simulink model "proxy"  (R2017b)
settings: Solver=ode3  StartTime=0.0  StopTime=inf  FixedStep=0.01  RelTol=1e-3  EnableMultiTasking=on
model workspace (MAT data in the model file):
  SL_ROS_VariableLengthArrays_MaxSizes.CommonInfo.ArrayTruncateAction = 'EmitWarning'
  SL_ROS_VariableLengthArrays_MaxSizes.MsgTypeMap = containers.Map
  SL_ROS_VariableLengthArrays_MaxSizes.MsgTypeMap.serialization.keys = {'std_msgs/Float32MultiArray'}
  SL_ROS_VariableLengthArrays_MaxSizes.MsgTypeMap.serialization.values{1}.PropertyName = 'Data'
  SL_ROS_VariableLengthArrays_MaxSizes.MsgTypeMap.serialization.values{1}.DataType = 'single'
  SL_ROS_VariableLengthArrays_MaxSizes.MsgTypeMap.serialization.values{1}.MaxLength = 2
  SL_ROS_VariableLengthArrays_MaxSizes.MsgTypeMap.serialization.uniformity = 0
  SL_ROS_VariableLengthArrays_MaxSizes.MsgTypeMap.serialization.keyType = 'char'
  SL_ROS_VariableLengthArrays_MaxSizes.MsgTypeMap.serialization.valueType = 'any'
values from neighbouring files (symbols this model uses):
  filt = c2d(filt,sampleTime)    [Connect.m]
libraries: robotlib x8, simulink x6, simulink_extras x3, dspnetwork x3, etargetslib x2, xpcutilitieslib x1
(part 1 of 4)
settings Model: Creator=Centauro  LastModifiedBy=BCI-USER
settings DataIOCC: LimitDataPoints=on  SaveFormat=Array
settings OptimizationCC: PassReuseOutputArgsThreshold=0  MaxStackSize=64
settings DebuggingCC: ParameterTunabilityLossMsg=error  SFUnexpectedBacktrackingDiag=warning  SFNoUnconditionalDefaultTransitionDiag=warning  SFExecutionAtInitializationDiag=none
settings HardwareCC: ProdBitPerPointer=32  ProdBitPerSizeT=32  ProdBitPerPtrDiffT=32  ProdLargestAtomicFloat=None  ProdIntDivRoundTo=Undefined  ProdEndianess=Unspecified  ProdWordSize=32  ProdHWDeviceType=Generic->Unspecified (assume 32-bit Generic)  UseEmbeddedCoderFeatures=off
settings ModelReferenceCC: PropagateSignalLabelsOutOfModel=off
settings SFSimCC: MATLABDynamicMemAlloc=off
settings RTWCC: SystemTargetFile=ert.tlc  HardwareBoard=Robot Operating System (ROS)  TemplateMakefile=ert_default_tmf  GenerateReport=on  Toolchain=Catkin  LaunchReport=on  TargetLang=C++
settings CodeAppCC: ForceParamTrailComments=on  OperatorAnnotations=on
settings ERTTargetCC: ERTCustomFileBanners=off  SupportContinuousTime=on  SupportNonInlinedSFcns=on  RemoveResetFunc=off  ModelStepFunctionPrototypeControlCompliant=off
settings ConfigComp: CovMetricSettings=dw  CovHtmlReporting=on  CovSaveCumulativeToWorkspaceVar=on  CovSaveSingleToWorkspaceVar=on  CovExternalEMLEnable=off

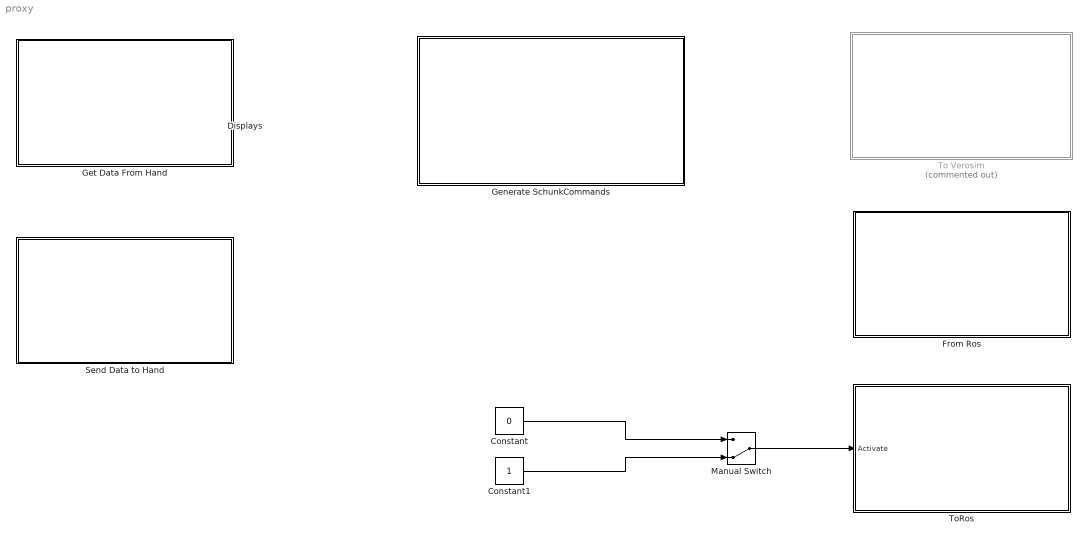
== system proxy ==
  Constant : Constant  Value=0  OutDataTypeStr=boolean
  Constant1 : Constant  OutDataTypeStr=boolean
  "Displays " : Subsystem
  From Ros : Subsystem
  "Generate SchunkCommands " : Subsystem
  Get Data From Hand : Subsystem
  Manual Switch : ManualSwitch  CurrentSetting=0
  Send Data to Hand : Subsystem
  To Verosim : Subsystem  Commented=on
  ToRos : Subsystem
  wires:
  Manual Switch/1 -> ToRos/1(Activate)
  Constant/1 -> Manual Switch/1
  Constant1/1 -> Manual Switch/2

== system proxy/Displays  ==
  Display{,1..3} (4 alike) : Display
  wires:
  [Forces] -> Display1/1
  [RotativePot] -> Display3/1
  [Header] -> Display/1
  [MotorsPot] -> Display2/1

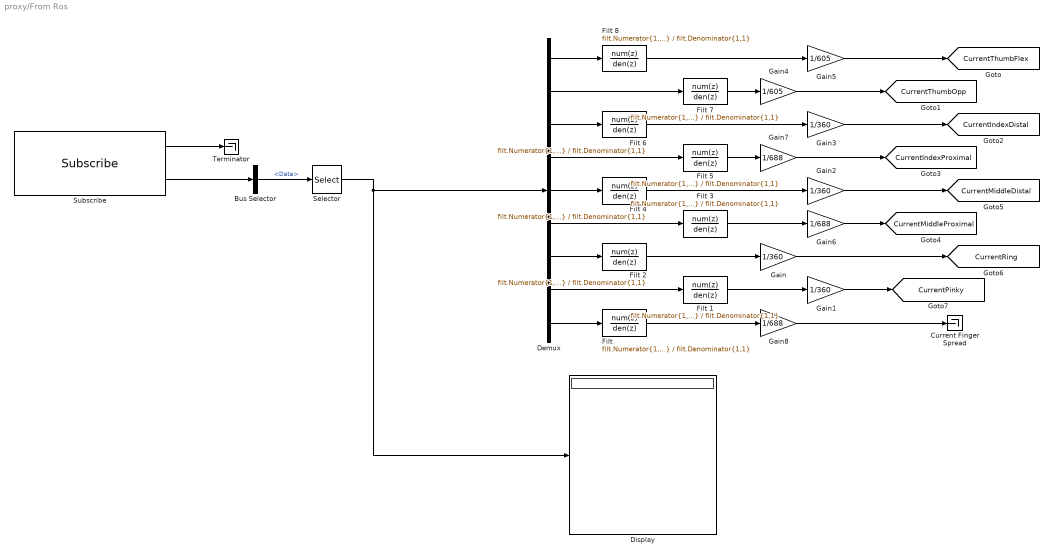
== system proxy/From Ros ==
  Bus Selector : BusSelector  OutputSignals=Data
  Current Finger Spread : Terminator
  Demux : Demux  Outputs=9
  Display : Display
  Filt {,1..8} (9 alike) : DiscreteTransferFcn  Numerator=filt.Numerator{1,1}  Denominator=filt.Denominator{1,1}  SampleTime=0.01
  Gain{,1..3} (4 alike) : Gain  Gain=1/360
  Gain4 : Gain  Gain=1/605
  Gain5 : Gain  Gain=1/605
  Gain6 : Gain  Gain=1/688
  Gain7 : Gain  Gain=1/688
  Gain8 : Gain  Gain=1/688
  Selector : Selector  IndexOptions=Index vector (dialog)  Indices=[1 2 3 4 5 6 7 8 9]  OutputSizes=1
  Subscribe : robotlib/Subscribe  SourceLibraryInfo=This block requires Robotics System Toolbox  topicSource=Select from ROS network  topic=/svh_controller/channel_currents  messageType=std_msgs/Float64MultiArray  sampleTime=0.01  messageQueueLength=1
      settings: SourceProductBaseCode=RO
  Terminator : Terminator
  tag scope: CurrentIndexDistal=global, CurrentIndexProximal=global, CurrentMiddleDistal=global, CurrentMiddleProximal=global, CurrentPinky=global, CurrentRing=global, CurrentThumbFlex=global, CurrentThumbOpp=global
  wires:
  Subscribe/1 -> Terminator/1
  Subscribe/2 -> Bus Selector/1
  Bus Selector/1 -> Selector/1  "<Data>"
  Selector/1 -> Demux/1, Display/1
  Demux/1 -> Filt 8/1
  Demux/2 -> Filt 7/1
  Demux/3 -> Filt 6/1
  Demux/4 -> Filt 5/1
  Demux/6 -> Filt 3/1
  Demux/5 -> Filt 4/1
  Demux/7 -> Filt 2/1
  Demux/8 -> Filt 1/1
  Demux/9 -> "Filt "/1
  "Filt "/1 -> Gain8/1
  Filt 1/1 -> Gain1/1
  Filt 2/1 -> Gain/1
  Filt 4/1 -> Gain2/1
  Filt 5/1 -> Gain7/1
  Filt 6/1 -> Gain3/1
  Filt 7/1 -> Gain4/1
  Filt 8/1 -> Gain5/1
  Gain1/1 -> [CurrentPinky]
  Gain/1 -> [CurrentRing]
  Filt 3/1 -> Gain6/1
  Gain2/1 -> [CurrentMiddleDistal]
  Gain3/1 -> [CurrentIndexDistal]
  Gain5/1 -> [CurrentThumbFlex]
  Gain4/1 -> [CurrentThumbOpp]
  Gain7/1 -> [CurrentIndexProximal]
  Gain6/1 -> [CurrentMiddleProximal]
  Gain8/1 -> Current Finger Spread/1

== system proxy/Generate SchunkCommands  ==
  Finger Spread : Subsystem
  Index Finger : Subsystem
  Middle Finger : Subsystem
  Pinky : Subsystem
  "Ring " : Subsystem
  Thumb : Subsystem

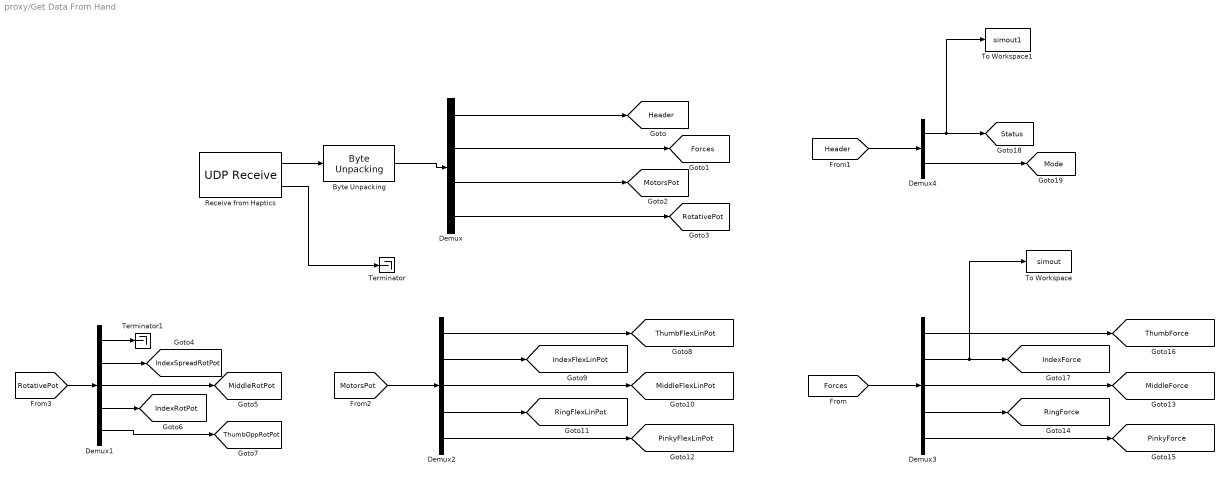
== system proxy/Get Data From Hand ==
  "Byte Unpacking " : xpcutilitieslib/Byte Unpacking   MaskUnpackedDataTypes={'single'}  MaskUnpackedDataSizes={[17]}  MaskAlignment=1
      settings: SourceProductName=Simulink Real-Time  SourceProductBaseCode=XP
  Demux : Demux  Outputs=[2, 5, 5, 5]
  Demux1 : Demux  Outputs=5
  Demux2 : Demux  Outputs=5
  Demux3 : Demux  Outputs=5
  Demux4 : Demux  Outputs=2
  Receive from Haptics : dspnetwork/UDP Receive  localURL='0.0.0.0'  localPort=15001  remoteURL='10.100.39.144'  remotePort=-1  recvBufferSize=17*4  dims=17*4  signalDatatype=uint8  isVarSize=off  showBlockingTime=on  blockingTime=inf  sampletime=0.01  blockPlatform=HOST
      settings: SourceProductName=DSP System Toolbox  SourceProductBaseCode=DS
  Terminator : Terminator
  Terminator1 : Terminator
  To Workspace : ToWorkspace  VariableName=simout  SaveFormat=Timeseries  SampleTime=-1
  To Workspace1 : ToWorkspace  VariableName=simout1  SaveFormat=Timeseries  SampleTime=-1
  tag scope: Forces=global, Header=global, IndexFlexLinPot=global, IndexForce=global, IndexRotPot=global, IndexSpreadRotPot=global, MiddleFlexLinPot=global, MiddleForce=global, MiddleRotPot=global, Mode=global, MotorsPot=global, PinkyFlexLinPot=global, PinkyForce=global, RingFlexLinPot=global, RingForce=global, RotativePot=global, Status=global, ThumbFlexLinPot=global, ThumbForce=global, ThumbOppRotPot=global
  wires:
  Demux/3 -> [MotorsPot]
  Demux/1 -> [Header]
  Demux/4 -> [RotativePot]
  Demux/2 -> [Forces]
  "Byte Unpacking "/1 -> Demux/1
  Receive from Haptics/1 -> "Byte Unpacking "/1
  Receive from Haptics/2 -> Terminator/1
  [RotativePot] -> Demux1/1
  Demux1/2 -> [IndexSpreadRotPot]
  Demux1/3 -> [MiddleRotPot]
  Demux1/4 -> [IndexRotPot]
  Demux1/5 -> [ThumbOppRotPot]
  Demux1/1 -> Terminator1/1
  Demux2/1 -> [ThumbFlexLinPot]
  Demux2/2 -> [IndexFlexLinPot]
  [MotorsPot] -> Demux2/1
  Demux2/3 -> [MiddleFlexLinPot]
  Demux2/4 -> [RingFlexLinPot]
  Demux2/5 -> [PinkyFlexLinPot]
  Demux3/1 -> [ThumbForce]
  Demux3/2 -> To Workspace/1, [IndexForce]
  [Forces] -> Demux3/1
  Demux3/3 -> [MiddleForce]
  Demux3/4 -> [RingForce]
  Demux3/5 -> [PinkyForce]
  [Header] -> Demux4/1
  Demux4/1 -> To Workspace1/1, [Status]
  Demux4/2 -> [Mode]

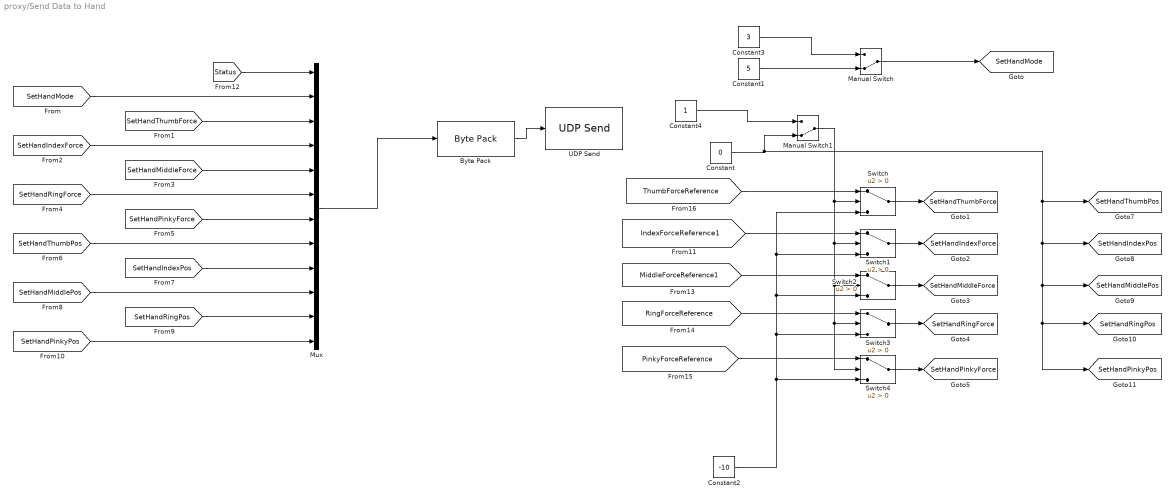
== system proxy/Send Data to Hand ==
  Byte Pack : etargetslib/Byte Pack  datatypes={'single'}  byteAlign=1
  Constant : Constant  Value=0  OutDataTypeStr=single
  Constant1 : Constant  Value=5  OutDataTypeStr=single
  Constant2 : Constant  Value=-10  OutDataTypeStr=single
  Constant3 : Constant  Value=3  OutDataTypeStr=single
  Constant4 : Constant  OutDataTypeStr=single
  Manual Switch : ManualSwitch  CurrentSetting=0
  Manual Switch1 : ManualSwitch  CurrentSetting=0
  Mux : Mux  Inputs=12
  Switch : Switch  Criteria=u2 > Threshold
  Switch1 : Switch  Criteria=u2 > Threshold
  Switch2 : Switch  Criteria=u2 > Threshold
  Switch3 : Switch  Criteria=u2 > Threshold  OutDataTypeStr=single
  Switch4 : Switch  Criteria=u2 > Threshold  OutDataTypeStr=single
  UDP Send : dspnetwork/UDP Send  remoteURL='10.100.39.144'  remotePort=12000  localURL='0.0.0.0'  localPortSource=Automatically determine  localPort=-1  sampletime=-1  blockPlatform=HOST  separateLengthPort=0
      settings: SourceProductName=DSP System Toolbox  SourceProductBaseCode=DS
  tag scope: SetHandIndexForce=global, SetHandIndexPos=global, SetHandMiddleForce=global, SetHandMiddlePos=global, SetHandMode=global, SetHandPinkyForce=global, SetHandPinkyPos=global, SetHandRingForce=global, SetHandRingPos=global, SetHandThumbForce=global, SetHandThumbPos=global
  wires:
  Byte Pack/1 -> UDP Send/1
  [SetHandMode] -> Mux/2
  Constant2/1 -> Switch4/3, Switch3/3, Switch2/3, Switch1/3, Switch/3
  [SetHandThumbForce] -> Mux/3
  [SetHandIndexForce] -> Mux/4
  [SetHandRingForce] -> Mux/6
  [SetHandMiddleForce] -> Mux/5
  [SetHandPinkyForce] -> Mux/7
  [SetHandThumbPos] -> Mux/8
  [SetHandIndexPos] -> Mux/9
  [SetHandMiddlePos] -> Mux/10
  [SetHandRingPos] -> Mux/11
  [SetHandPinkyPos] -> Mux/12
  Manual Switch/1 -> [SetHandMode]
  Constant1/1 -> Manual Switch/2
  Constant3/1 -> Manual Switch/1
  [Status] -> Mux/1
  Constant4/1 -> Manual Switch1/1
  Switch/1 -> [SetHandThumbForce]
  Manual Switch1/1 -> Switch2/2, Switch3/2, Switch4/2, Switch1/2, Switch/2
  Switch3/1 -> [SetHandRingForce]
  Switch4/1 -> [SetHandPinkyForce]
  [ThumbForceReference] -> Switch/1
  [IndexForceReference1] -> Switch1/1
  [MiddleForceReference1] -> Switch2/1
  [RingForceReference] -> Switch3/1
  [PinkyForceReference] -> Switch4/1
  Switch2/1 -> [SetHandMiddleForce]
  Switch1/1 -> [SetHandIndexForce]
  Constant/1 -> [SetHandThumbPos], [SetHandIndexPos], [SetHandMiddlePos], [SetHandRingPos], [SetHandPinkyPos], Manual Switch1/2
  Mux/1 -> Byte Pack/1

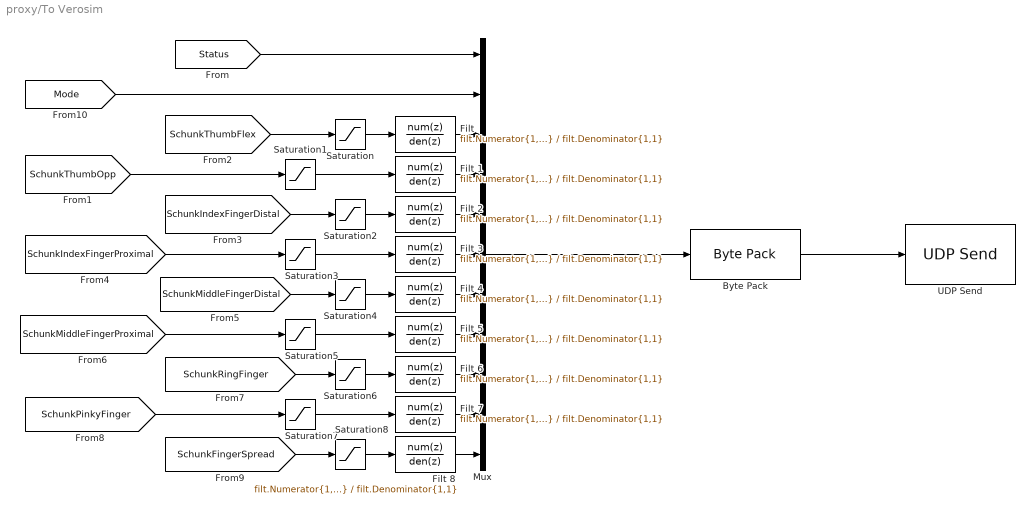
== system proxy/To Verosim ==
  Byte Pack : etargetslib/Byte Pack  datatypes={'single'}  byteAlign=1
  Filt {,1..8} (9 alike) : DiscreteTransferFcn  Numerator=filt.Numerator{1,1}  Denominator=filt.Denominator{1,1}  SampleTime=0.01
  Mux : Mux  Inputs=11
  Saturation : Saturate  UpperLimit=0.97  LowerLimit=0
  Saturation1 : Saturate  UpperLimit=0.99  LowerLimit=0
  Saturation2 : Saturate  UpperLimit=1.33  LowerLimit=0
  Saturation3 : Saturate  UpperLimit=0.80  LowerLimit=0
  Saturation4 : Saturate  UpperLimit=1.33  LowerLimit=0
  Saturation5 : Saturate  UpperLimit=0.80  LowerLimit=0
  Saturation6 : Saturate  UpperLimit=0.98  LowerLimit=0
  Saturation7 : Saturate  UpperLimit=0.98  LowerLimit=0
  Saturation8 : Saturate  UpperLimit=0.58  LowerLimit=0
  UDP Send : dspnetwork/UDP Send  remoteURL='10.100.39.22'  remotePort=15000  localURL='0.0.0.0'  localPortSource=Automatically determine  localPort=-1  sampletime=-1  blockPlatform=HOST  separateLengthPort=0
      settings: SourceProductName=DSP System Toolbox  SourceProductBaseCode=DS
  wires:
  [SchunkThumbOpp] -> Saturation1/1
  Byte Pack/1 -> UDP Send/1
  Mux/1 -> Byte Pack/1
  [SchunkThumbFlex] -> Saturation/1
  [SchunkIndexFingerDistal] -> Saturation2/1
  [SchunkIndexFingerProximal] -> Saturation3/1
  [SchunkMiddleFingerDistal] -> Saturation4/1
  [SchunkMiddleFingerProximal] -> Saturation5/1
  [SchunkRingFinger] -> Saturation6/1
  [SchunkPinkyFinger] -> Saturation7/1
  [SchunkFingerSpread] -> Saturation8/1
  Saturation/1 -> "Filt "/1
  Saturation1/1 -> Filt 1/1
  Saturation2/1 -> Filt 2/1
  Saturation3/1 -> Filt 3/1
  Saturation4/1 -> Filt 4/1
  Saturation5/1 -> Filt 5/1
  Saturation6/1 -> Filt 6/1
  Saturation7/1 -> Filt 7/1
  Saturation8/1 -> Filt 8/1
  [Mode] -> Mux/2
  [Status] -> Mux/1
  "Filt "/1 -> Mux/3
  Filt 1/1 -> Mux/4
  Filt 2/1 -> Mux/5
  Filt 3/1 -> Mux/6
  Filt 4/1 -> Mux/7
  Filt 5/1 -> Mux/8
  Filt 6/1 -> Mux/9
  Filt 7/1 -> Mux/10
  Filt 8/1 -> Mux/11

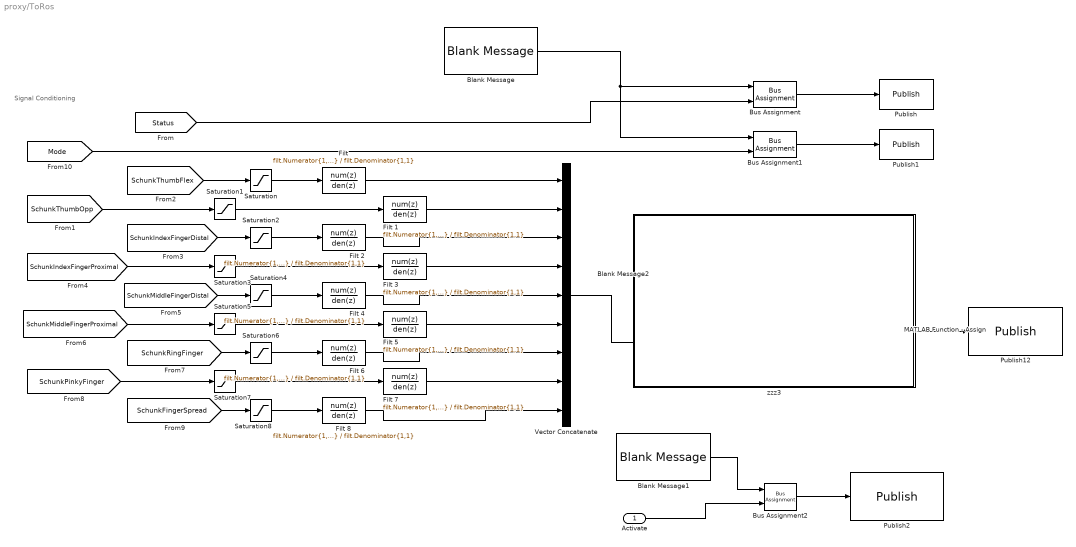
== system proxy/ToRos ==
  note: Signal Conditioning
  Activate : Inport
  Blank Message : robotlib/Blank Message  SourceLibraryInfo=This block requires Robotics System Toolbox  messageType=std_msgs/Float32  SampleTime=0.01
      settings: SourceProductBaseCode=RO
  Blank Message1 : robotlib/Blank Message  SourceLibraryInfo=This block requires Robotics System Toolbox  messageType=std_msgs/Bool  SampleTime=inf
      settings: SourceProductBaseCode=RO
  Blank Message2 : robotlib/Blank Message  SourceLibraryInfo=This block requires Robotics System Toolbox  messageType=sensor_msgs/JointState  SampleTime=inf
      settings: SourceProductBaseCode=RO
  Bus Assignment : BusAssignment  AssignedSignals=Data
  Bus Assignment1 : BusAssignment  AssignedSignals=Data
  Bus Assignment2 : BusAssignment  AssignedSignals=Data
  Filt {,1..8} (9 alike) : DiscreteTransferFcn  Numerator=filt.Numerator{1,1}  Denominator=filt.Denominator{1,1}  SampleTime=0.01
  MATLAB Function - Assign : MATLAB Function  TreatAsAtomicUnit=on
  Publish : robotlib/Publish  SourceLibraryInfo=This block requires Robotics System Toolbox  topicSource=Specify your own  topic=/MatlabStatus  messageType=std_msgs/Float32  messageQueueLength=1
      settings: SourceProductBaseCode=RO
  Publish1 : robotlib/Publish  SourceLibraryInfo=This block requires Robotics System Toolbox  topicSource=Specify your own  topic=/MatlabMode  messageType=std_msgs/Float32  messageQueueLength=1
      settings: SourceProductBaseCode=RO
  Publish12 : robotlib/Publish  SourceLibraryInfo=This block requires Robotics System Toolbox  topicSource=Specify your own  topic=/scan  messageType=sensor_msgs/JointState  messageQueueLength=1
      settings: SourceProductBaseCode=RO
  Publish2 : robotlib/Publish  SourceLibraryInfo=This block requires Robotics System Toolbox  topicSource=Select from ROS network  topic=/trigger_exo_hand  messageType=std_msgs/Bool  messageQueueLength=1
      settings: SourceProductBaseCode=RO
  Saturation : Saturate  UpperLimit=0.97  LowerLimit=0
  Saturation1 : Saturate  UpperLimit=0.99  LowerLimit=0
  Saturation2 : Saturate  UpperLimit=1.33  LowerLimit=0
  Saturation3 : Saturate  UpperLimit=0.80  LowerLimit=0
  Saturation4 : Saturate  UpperLimit=1.33  LowerLimit=0
  Saturation5 : Saturate  UpperLimit=0.80  LowerLimit=0
  Saturation6 : Saturate  UpperLimit=0.98  LowerLimit=0
  Saturation7 : Saturate  UpperLimit=0.98  LowerLimit=0
  Saturation8 : Saturate  UpperLimit=0.58  LowerLimit=0.20
  Vector Concatenate : Concatenate  NumInputs=9
  zzz3 : Subsystem  TreatAsAtomicUnit=on
      settings: OpenFcn=% no-op
      mask Display: disp('')
  wires:
  Bus Assignment/1 -> Publish/1
  Blank Message/1 -> Bus Assignment1/1, Bus Assignment/1
  Bus Assignment1/1 -> Publish1/1
  Vector Concatenate/1 -> MATLAB Function - Assign/2(u)
  Blank Message2/1 -> MATLAB Function - Assign/1(blankMessage)
  MATLAB Function - Assign/1(msg) -> Publish12/1
  "Filt "/1 -> Vector Concatenate/1
  Filt 5/1 -> Vector Concatenate/6
  Filt 6/1 -> Vector Concatenate/7
  Filt 3/1 -> Vector Concatenate/4
  Filt 2/1 -> Vector Concatenate/3
  Filt 4/1 -> Vector Concatenate/5
  Filt 8/1 -> Vector Concatenate/9
  Filt 1/1 -> Vector Concatenate/2
  Filt 7/1 -> Vector Concatenate/8
  [Status] -> Bus Assignment/2
  [Mode] -> Bus Assignment1/2
  Saturation/1 -> "Filt "/1
  Saturation6/1 -> Filt 6/1
  [SchunkMiddleFingerDistal] -> Saturation4/1
  [SchunkIndexFingerProximal] -> Saturation3/1
  [SchunkThumbFlex] -> Saturation/1
  [SchunkFingerSpread] -> Saturation8/1
  Saturation1/1 -> Filt 1/1
  [SchunkPinkyFinger] -> Saturation7/1
  Saturation3/1 -> Filt 3/1
  [SchunkMiddleFingerProximal] -> Saturation5/1
  [SchunkIndexFingerDistal] -> Saturation2/1
  Saturation5/1 -> Filt 5/1
  [SchunkThumbOpp] -> Saturation1/1
  Saturation4/1 -> Filt 4/1
  [SchunkRingFinger] -> Saturation6/1
  Saturation7/1 -> Filt 7/1
  Saturation8/1 -> Filt 8/1
  Saturation2/1 -> Filt 2/1
  Blank Message1/1 -> Bus Assignment2/1
  Bus Assignment2/1 -> Publish2/1
  Activate/1 -> Bus Assignment2/2

== system proxy/Generate SchunkCommands /Finger Spread ==
  Display : Display
  MATLAB Function : MATLAB Function  TreatAsAtomicUnit=on
  tag scope: SchunkFingerSpread=global
  wires:
  [IndexSpreadRotPot] -> Display/1, MATLAB Function/1(u)
  MATLAB Function/1(y) -> [SchunkFingerSpread]

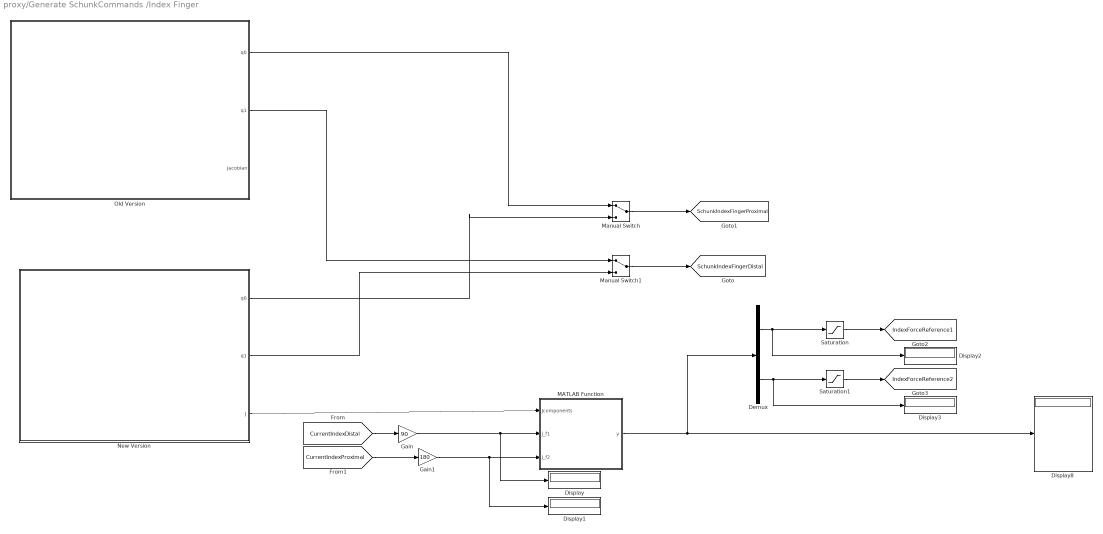
== system proxy/Generate SchunkCommands /Index Finger ==
  Demux : Demux  Outputs=2
  Display{,1..3,8} (5 alike) : Display
  Gain : Gain  Gain=90
  Gain1 : Gain  Gain=180
  MATLAB Function : MATLAB Function  TreatAsAtomicUnit=on
  Manual Switch : ManualSwitch
  Manual Switch1 : ManualSwitch
  New Version : Subsystem
  Old Version : Subsystem
  Saturation : Saturate  UpperLimit=5  LowerLimit=-5
  Saturation1 : Saturate  UpperLimit=5  LowerLimit=-5
  tag scope: IndexForceReference1=global, IndexForceReference2=global, SchunkIndexFingerDistal=global, SchunkIndexFingerProximal=global
  wires:
  MATLAB Function/1(y) -> Demux/1, Display8/1
  Manual Switch1/1 -> [SchunkIndexFingerDistal]
  Old Version/2(q1) -> Manual Switch1/1
  Manual Switch/1 -> [SchunkIndexFingerProximal]
  Old Version/1(q0) -> Manual Switch/1
  New Version/3(J) -> MATLAB Function/1(Jcomponents)
  New Version/1(q0) -> Manual Switch/2
  New Version/2(q1) -> Manual Switch1/2
  Demux/1 -> Display2/1, Saturation/1
  Demux/2 -> Display3/1, Saturation1/1
  [CurrentIndexDistal] -> Gain/1
  [CurrentIndexProximal] -> Gain1/1
  Saturation1/1 -> [IndexForceReference2]
  Saturation/1 -> [IndexForceReference1]
  Gain1/1 -> Display1/1, MATLAB Function/3(j_f2)
  Gain/1 -> Display/1, MATLAB Function/2(j_f1)

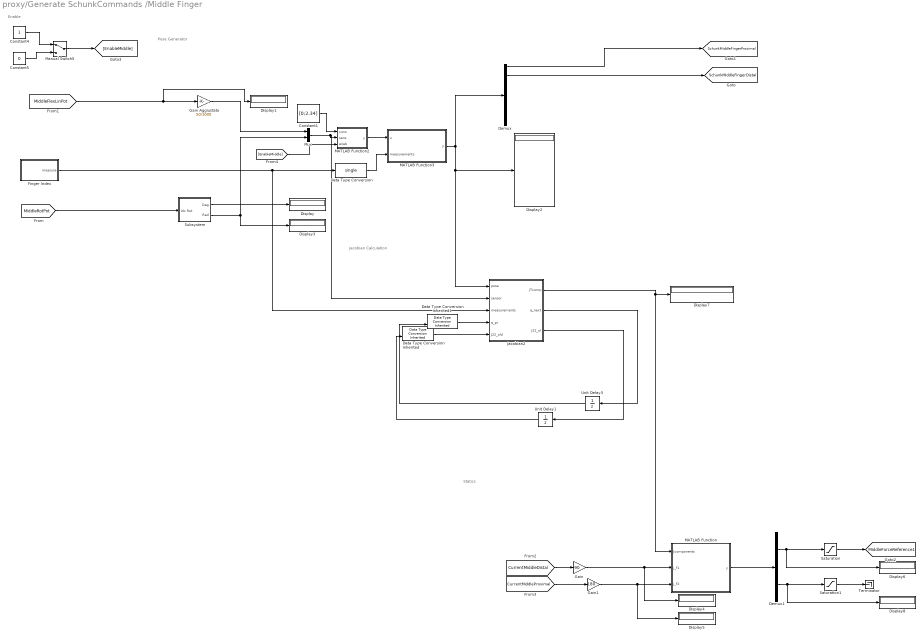
== system proxy/Generate SchunkCommands /Middle Finger ==
  note: Enable
  note: Statics
  note: Jacobian Calculation
  note: Pose Generator
  Constant1 : Constant  Value=[0;2.34]  OutDataTypeStr=single
  Constant4 : Constant  OutDataTypeStr=single
  Constant5 : Constant  Value=0  OutDataTypeStr=single
  Data Type Conversion Inherited : simulink/Signal Attributes/Data Type Conversion Inherited  ConvertRealWorld=Real World Value  DoSatur=off
      settings: SourceProductName=Simulink  SourceProductBaseCode=SL
  Data Type Conversion Inherited1 : simulink/Signal Attributes/Data Type Conversion Inherited  ConvertRealWorld=Real World Value  DoSatur=off
      settings: SourceProductName=Simulink  SourceProductBaseCode=SL
  Data Type Conversion : DataTypeConversion  OutDataTypeStr=single
  Demux : Demux  Outputs=8
  Demux1 : Demux  Outputs=2
  Display{,1..8} (9 alike) : Display
  "Finger Index " : Subsystem
  Gain : Gain  Gain=90
  Gain Aggiustato : Gain  Gain=50/1000
  Gain1 : Gain  Gain=180
  Jacobian2 : MATLAB Function  TreatAsAtomicUnit=on  SystemSampleTime=0.01
  MATLAB Function : MATLAB Function  TreatAsAtomicUnit=on
  MATLAB Function2 : MATLAB Function  TreatAsAtomicUnit=on
  MATLAB Function3 : MATLAB Function  TreatAsAtomicUnit=on
  Manual Switch5 : ManualSwitch
  Mux : Mux  Inputs=2
  Saturation : Saturate  UpperLimit=5  LowerLimit=-5
  Saturation1 : Saturate  UpperLimit=5  LowerLimit=-5
  Subsystem : Subsystem
  Terminator : Terminator
  Unit Delay1 : UnitDelay  InitialCondition=-1  SampleTime=0.01
  Unit Delay3 : UnitDelay  InitialCondition=[0;2.3]  SampleTime=0.01
  tag scope: MiddleForceReference1=global, SchunkMiddleFingerDistal=global, SchunkMiddleFingerProximal=global
  wires:
  Demux/1 -> [SchunkMiddleFingerProximal]
  Demux/2 -> [SchunkMiddleFingerDistal]
  [MiddleRotPot] -> Subsystem/1(Idx Rot)
  Subsystem/1(Deg) -> Display/1
  Gain Aggiustato/1 -> Mux/1
  Constant1/1 -> MATLAB Function2/1(cons)
  Subsystem/2(Rad) -> Mux/2, Display3/1
  Data Type Conversion/1 -> MATLAB Function3/2(measurements)
  MATLAB Function2/1(y) -> MATLAB Function3/1(u)
  [MiddleFlexLinPot] -> Gain Aggiustato/1, Display1/1
  Unit Delay3/1 -> Data Type Conversion Inherited1/2
  Jacobian2/3(J22_ol) -> Unit Delay1/1
  Data Type Conversion Inherited/1 -> Jacobian2/5(J22_old)
  Mux/1 -> Jacobian2/2(sensor), MATLAB Function2/2(sens)
  Unit Delay1/1 -> Data Type Conversion Inherited/2
  "Finger Index "/1(measure) -> Jacobian2/3(measurements), Data Type Conversion/1
  Data Type Conversion Inherited1/1 -> Jacobian2/4(q_pr)
  Jacobian2/2(q_next) -> Unit Delay3/1
  MATLAB Function3/1(y) -> Jacobian2/1(pose), Display2/1, Demux/1
  [CurrentMiddleProximal] -> Gain1/1
  Gain/1 -> Display4/1, MATLAB Function/2(j_f1)
  [CurrentMiddleDistal] -> Gain/1
  Saturation1/1 -> Terminator/1
  Demux1/2 -> Display8/1, Saturation1/1
  Gain1/1 -> Display5/1, MATLAB Function/3(j_f2)
  Demux1/1 -> Display6/1, Saturation/1
  Jacobian2/1(JTcomp) -> MATLAB Function/1(Jcomponents), Display7/1
  MATLAB Function/1(y) -> Demux1/1
  Saturation/1 -> [MiddleForceReference1]
  Manual Switch5/1 -> [EnableMiddle]
  Constant5/1 -> Manual Switch5/2
  Constant4/1 -> Manual Switch5/1
  [EnableMiddle] -> MATLAB Function2/3(enab)

== system proxy/Generate SchunkCommands /Pinky ==
  note: Pose Estimation
  note: Statics
  Constant1 : Constant  Value=0  OutDataTypeStr=single
  Gain : Gain  Gain=5
  Manual Switch : ManualSwitch  CurrentSetting=0
  Pose Estimation : MATLAB Function  TreatAsAtomicUnit=on
  Saturation : Saturate  UpperLimit=950  LowerLimit=0
  Saturation1 : Saturate  UpperLimit=5  LowerLimit=-5
  tag scope: PinkyForceReference=global, SchunkPinkyFinger=global
  wires:
  [PinkyFlexLinPot] -> Saturation/1
  Saturation/1 -> Pose Estimation/1(u)
  Manual Switch/1 -> [SchunkPinkyFinger]
  Pose Estimation/1(y) -> Manual Switch/1
  Constant1/1 -> Manual Switch/2
  Gain/1 -> Saturation1/1
  [CurrentPinky] -> Gain/1
  Saturation1/1 -> [PinkyForceReference]

== system proxy/Generate SchunkCommands /Ring  ==
  note: Statics
  note: Pose Estimation
  Constant1 : Constant  Value=0  OutDataTypeStr=single
  Gain : Gain  Gain=5
  Manual Switch : ManualSwitch
  Pose Estimation : MATLAB Function  TreatAsAtomicUnit=on
  Saturation : Saturate  UpperLimit=950  LowerLimit=0
  Saturation1 : Saturate  UpperLimit=5  LowerLimit=-5
  tag scope: RingForceReference=global, SchunkRingFinger=global
  wires:
  [RingFlexLinPot] -> Saturation/1
  Constant1/1 -> Manual Switch/2
  Manual Switch/1 -> [SchunkRingFinger]
  Pose Estimation/1(y) -> Manual Switch/1
  Gain/1 -> Saturation1/1
  [CurrentRing] -> Gain/1
  Saturation1/1 -> [RingForceReference]
  Saturation/1 -> Pose Estimation/1(u)

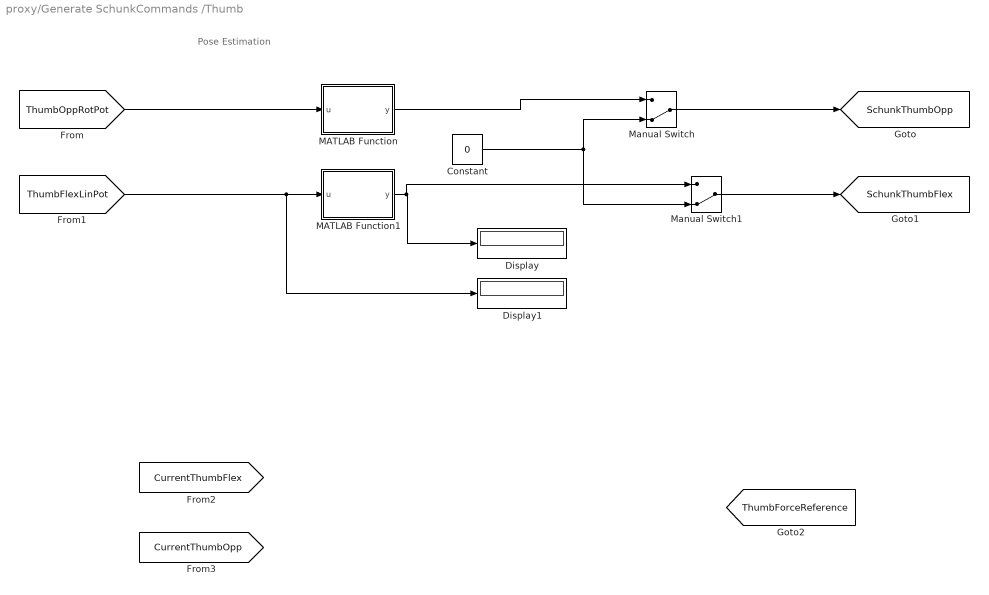
== system proxy/Generate SchunkCommands /Thumb ==
  note: Pose Estimation
  Constant : Constant  Value=0  OutDataTypeStr=single
  Display : Display
  Display1 : Display
  MATLAB Function : MATLAB Function  TreatAsAtomicUnit=on
  MATLAB Function1 : MATLAB Function  TreatAsAtomicUnit=on
  Manual Switch : ManualSwitch  CurrentSetting=0
  Manual Switch1 : ManualSwitch  CurrentSetting=0
  tag scope: SchunkThumbFlex=global, SchunkThumbOpp=global, ThumbForceReference=global
  wires:
  [ThumbOppRotPot] -> MATLAB Function/1(u)
  MATLAB Function1/1(y) -> Manual Switch1/1, Display/1
  [ThumbFlexLinPot] -> Display1/1, MATLAB Function1/1(u)
  Manual Switch/1 -> [SchunkThumbOpp]
  MATLAB Function/1(y) -> Manual Switch/1
  Manual Switch1/1 -> [SchunkThumbFlex]
  Constant/1 -> Manual Switch1/2, Manual Switch/2

== system proxy/ToRos/zzz3 ==

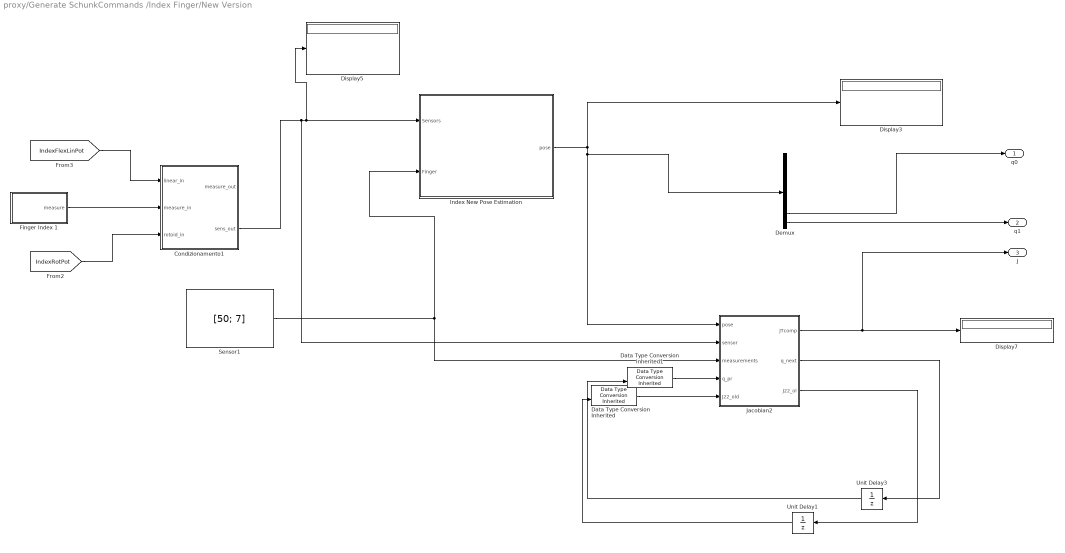
== system proxy/Generate SchunkCommands /Index Finger/New Version ==
  Condizionamento1 : Subsystem
  Data Type Conversion Inherited : simulink/Signal Attributes/Data Type Conversion Inherited  ConvertRealWorld=Real World Value  DoSatur=off
      settings: SourceProductName=Simulink  SourceProductBaseCode=SL
  Data Type Conversion Inherited1 : simulink/Signal Attributes/Data Type Conversion Inherited  ConvertRealWorld=Real World Value  DoSatur=off
      settings: SourceProductName=Simulink  SourceProductBaseCode=SL
  Demux : Demux  Outputs=8
  Display3 : Display
  Display5 : Display
  Display7 : Display
  Finger Index 1 : Subsystem
  "Index New Pose Estimation " : MATLAB Function  TreatAsAtomicUnit=on
  Jacobian2 : MATLAB Function  TreatAsAtomicUnit=on  SystemSampleTime=0.01
  Sensor1 : Constant  Value=[50; 7]
  Unit Delay1 : UnitDelay  InitialCondition=-1  SampleTime=0.01
  Unit Delay3 : UnitDelay  InitialCondition=[0;2.3]  SampleTime=0.01
  q0 : Outport
  q1 : Outport  Port=2
  J : Outport  Port=3
  wires:
  Unit Delay3/1 -> Data Type Conversion Inherited1/2
  Sensor1/1 -> Jacobian2/3(measurements), "Index New Pose Estimation "/2(Finger)
  Data Type Conversion Inherited1/1 -> Jacobian2/4(q_pr)
  Jacobian2/2(q_next) -> Unit Delay3/1
  [IndexRotPot] -> Condizionamento1/3(rotoid_in)
  Finger Index 1/1(measure) -> Condizionamento1/2(measure_in)
  [IndexFlexLinPot] -> Condizionamento1/1(linear_in)
  "Index New Pose Estimation "/1(pose) -> Demux/1, Jacobian2/1(pose), Display3/1
  Unit Delay1/1 -> Data Type Conversion Inherited/2
  Jacobian2/3(J22_ol) -> Unit Delay1/1
  Condizionamento1/2(sens_out) -> Jacobian2/2(sensor), Display5/1, "Index New Pose Estimation "/1(Sensors)
  Data Type Conversion Inherited/1 -> Jacobian2/5(J22_old)
  Jacobian2/1(JTcomp) -> J/1, Display7/1
  Demux/7 -> q0/1
  Demux/8 -> q1/1

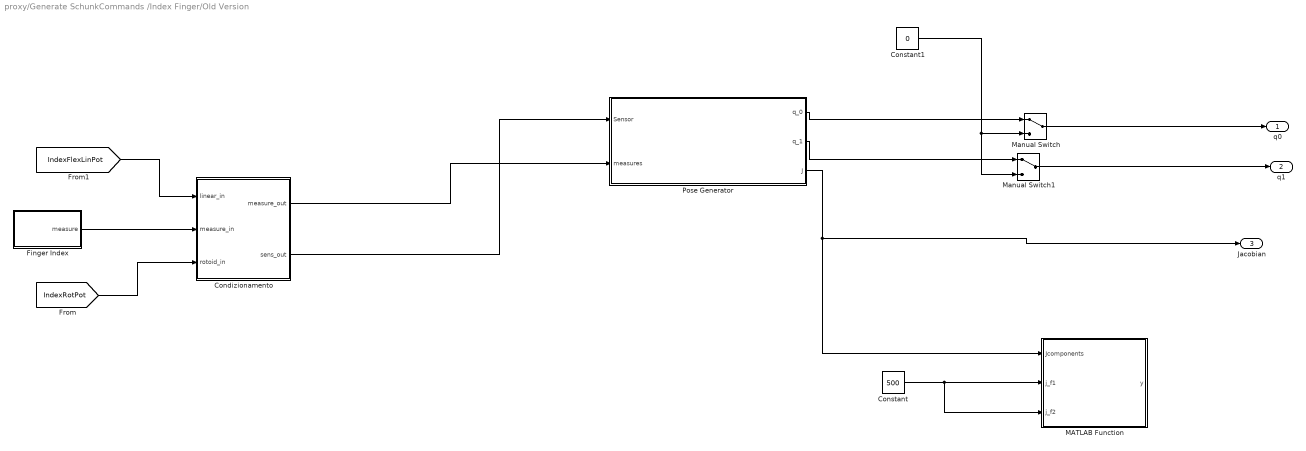
== system proxy/Generate SchunkCommands /Index Finger/Old Version ==
  Condizionamento : Subsystem
  Constant : Constant  Value=500  OutDataTypeStr=single
  Constant1 : Constant  Value=0  OutDataTypeStr=single
  "Finger Index " : Subsystem
  MATLAB Function : MATLAB Function  TreatAsAtomicUnit=on
  Manual Switch : ManualSwitch
  Manual Switch1 : ManualSwitch
  Pose Generator : Subsystem
  q0 : Outport
  q1 : Outport  Port=2
  Jacobian : Outport  Port=3
  wires:
  Constant/1 -> MATLAB Function/3(j_f2), MATLAB Function/2(j_f1)
  Pose Generator/2(q_1) -> Manual Switch1/1
  Manual Switch1/1 -> q1/1
  Constant1/1 -> Manual Switch1/2, Manual Switch/2
  Manual Switch/1 -> q0/1
  Pose Generator/1(q_0) -> Manual Switch/1
  Pose Generator/3(J) -> Jacobian/1, MATLAB Function/1(Jcomponents)
  Condizionamento/1(measure_out) -> Pose Generator/2(measures)
  [IndexRotPot] -> Condizionamento/3(rotoid_in)
  Condizionamento/2(sens_out) -> Pose Generator/1("Sensor ")
  "Finger Index "/1(measure) -> Condizionamento/2(measure_in)
  [IndexFlexLinPot] -> Condizionamento/1(linear_in)

== system proxy/Generate SchunkCommands /Middle Finger/Finger Index  ==
  Mux1 : Mux  Inputs=2
  finger width : Constant  Value=7
  proximal length : Constant  Value=50
  measure : Outport
  wires:
  Mux1/1 -> measure/1
  finger width/1 -> Mux1/1
  proximal length/1 -> Mux1/2

== system proxy/Generate SchunkCommands /Middle Finger/Subsystem ==
  Idx Rot : Inport
  Constant : Constant  Value=2*pi - 10*pi/180 - pi/2  OutDataTypeStr=single
  Gain Vero : Gain  Commented=through  Gain=330/1024
  Gain Aggiustato : Gain  Gain=350*pi/(1024*180)
  Radians to Degrees : simulink_extras/Transformations/Radians to Degrees
  Sum1 : Sum  Inputs=|-+
  Deg : Outport
  Rad : Outport  Port=2
  wires:
  Idx Rot/1 -> Gain Vero/1
  Radians to Degrees/1 -> Deg/1
  Gain Vero/1 -> Gain Aggiustato/1
  Constant/1 -> Sum1/2
  Gain Aggiustato/1 -> Sum1/1
  Sum1/1 -> Radians to Degrees/1, Rad/1

== system proxy/Generate SchunkCommands /Index Finger/New Version/Condizionamento1 ==
  linear_in : Inport
  measure_in : Inport  Port=2
  rotoid_in : Inport  Port=3
  Data Type Conversion : DataTypeConversion  OutDataTypeStr=single
  Display : Display
  Display1 : Display
  Gain Aggiustato : Gain  Gain=50/1000
  Mux : Mux  Inputs=2
  Subsystem : Subsystem
  measure_out : Outport
  sens_out : Outport  Port=2
  wires:
  linear_in/1 -> Gain Aggiustato/1
  Subsystem/1(Deg) -> Display/1
  Gain Aggiustato/1 -> Mux/1
  Data Type Conversion/1 -> measure_out/1
  measure_in/1 -> Data Type Conversion/1
  Subsystem/2(Rad) -> Mux/2, Display1/1
  rotoid_in/1 -> Subsystem/1(Idx Rot)
  Mux/1 -> sens_out/1

== system proxy/Generate SchunkCommands /Index Finger/New Version/Finger Index 1 ==
  Mux1 : Mux  Inputs=2
  finger width : Constant  Value=10
  proximal length : Constant  Value=50
  measure : Outport
  wires:
  Mux1/1 -> measure/1
  finger width/1 -> Mux1/1
  proximal length/1 -> Mux1/2

== system proxy/Generate SchunkCommands /Index Finger/Old Version/Condizionamento ==
  linear_in : Inport
  measure_in : Inport  Port=2
  rotoid_in : Inport  Port=3
  Data Type Conversion : DataTypeConversion  OutDataTypeStr=single
  Display : Display
  Display1 : Display
  Gain Aggiustato : Gain  Gain=50/1000
  Mux : Mux  Inputs=2
  Subsystem : Subsystem
  measure_out : Outport
  sens_out : Outport  Port=2
  wires:
  linear_in/1 -> Gain Aggiustato/1
  Subsystem/1(Deg) -> Display/1
  Gain Aggiustato/1 -> Mux/1
  Data Type Conversion/1 -> measure_out/1
  measure_in/1 -> Data Type Conversion/1
  Subsystem/2(Rad) -> Mux/2, Display1/1
  rotoid_in/1 -> Subsystem/1(Idx Rot)
  Mux/1 -> sens_out/1

== system proxy/Generate SchunkCommands /Index Finger/Old Version/Finger Index  ==
  Mux1 : Mux  Inputs=2
  finger width : Constant  Value=10
  proximal length : Constant  Value=50
  measure : Outport
  wires:
  Mux1/1 -> measure/1
  finger width/1 -> Mux1/1
  proximal length/1 -> Mux1/2

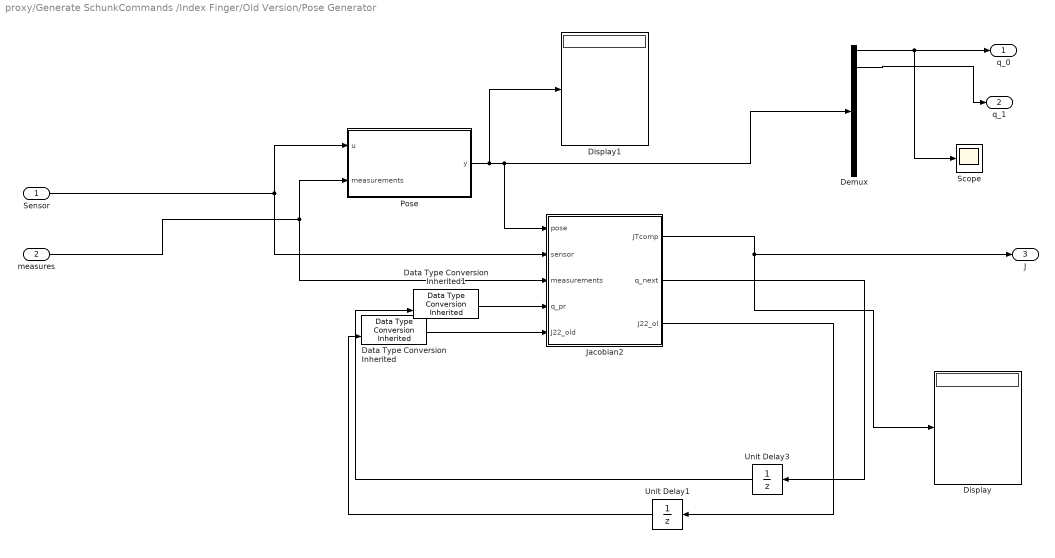
== system proxy/Generate SchunkCommands /Index Finger/Old Version/Pose Generator ==
  "Sensor " : Inport
  measures : Inport  Port=2
  Data Type Conversion Inherited : simulink/Signal Attributes/Data Type Conversion Inherited  ConvertRealWorld=Real World Value  DoSatur=off
      settings: SourceProductName=Simulink  SourceProductBaseCode=SL
  Data Type Conversion Inherited1 : simulink/Signal Attributes/Data Type Conversion Inherited  ConvertRealWorld=Real World Value  DoSatur=off
      settings: SourceProductName=Simulink  SourceProductBaseCode=SL
  Demux : Demux  Outputs=8
  Display : Display
  Display1 : Display
  Jacobian2 : MATLAB Function  TreatAsAtomicUnit=on  SystemSampleTime=0.01
  Pose : MATLAB Function  TreatAsAtomicUnit=on
  Scope : Scope
  Unit Delay1 : UnitDelay  InitialCondition=-1  SampleTime=0.01
  Unit Delay3 : UnitDelay  InitialCondition=[0;2.3]  SampleTime=0.01
  q_0 : Outport
  q_1 : Outport  Port=2
  J : Outport  Port=3
  wires:
  Demux/1 -> Scope/1, q_0/1
  Demux/2 -> q_1/1
  Jacobian2/1(JTcomp) -> J/1, Display/1
  Jacobian2/2(q_next) -> Unit Delay3/1
  Jacobian2/3(J22_ol) -> Unit Delay1/1
  Pose/1(y) -> Display1/1, Jacobian2/1(pose), Demux/1
  measures/1 -> Jacobian2/3(measurements), Pose/2(measurements)
  "Sensor "/1 -> Jacobian2/2(sensor), Pose/1(u)
  Unit Delay1/1 -> Data Type Conversion Inherited/2
  Data Type Conversion Inherited/1 -> Jacobian2/5(J22_old)
  Data Type Conversion Inherited1/1 -> Jacobian2/4(q_pr)
  Unit Delay3/1 -> Data Type Conversion Inherited1/2

== system proxy/Generate SchunkCommands /Index Finger/New Version/Condizionamento1/Subsystem ==
  Idx Rot : Inport
  Constant : Constant  Value=2*pi - 20*pi/180 - pi/2  OutDataTypeStr=single
  Gain Vero : Gain  Commented=through  Gain=330/1024
  Gain Aggiustato : Gain  Gain=350*pi/(1024*180)
  Radians to Degrees : simulink_extras/Transformations/Radians to Degrees
  Sum1 : Sum  Inputs=|-+
  Deg : Outport
  Rad : Outport  Port=2
  wires:
  Idx Rot/1 -> Gain Vero/1
  Radians to Degrees/1 -> Deg/1
  Gain Vero/1 -> Gain Aggiustato/1
  Constant/1 -> Sum1/2
  Gain Aggiustato/1 -> Sum1/1
  Sum1/1 -> Radians to Degrees/1, Rad/1

== system proxy/Generate SchunkCommands /Index Finger/Old Version/Condizionamento/Subsystem ==
  Idx Rot : Inport
  Constant : Constant  Value=2*pi - 10*pi/180 - pi/2  OutDataTypeStr=single
  Gain Vero : Gain  Commented=through  Gain=330/1024
  Gain Aggiustato : Gain  Gain=350*pi/(1024*180)
  Radians to Degrees : simulink_extras/Transformations/Radians to Degrees
  Sum1 : Sum  Inputs=|-+
  Deg : Outport
  Rad : Outport  Port=2
  wires:
  Idx Rot/1 -> Gain Vero/1
  Radians to Degrees/1 -> Deg/1
  Gain Vero/1 -> Gain Aggiustato/1
  Constant/1 -> Sum1/2
  Gain Aggiustato/1 -> Sum1/1
  Sum1/1 -> Radians to Degrees/1, Rad/1

== matlab function proxy/Generate SchunkCommands /Finger Spread/MATLAB Function ==
  data: u input; y output
function y = fcn(u)
%#codegen
y = (((-u + 460)/50)/2);

== matlab function proxy/Generate SchunkCommands /Thumb/MATLAB Function ==
  data: u input; y output
function y = fcn(u)
%#codegen

y = (u - 380) / 220;

== matlab function proxy/Generate SchunkCommands /Thumb/MATLAB Function1 ==
  data: u input; y output
function y = fcn(u)
%#codegen

y = single( (u - 0) / 400);

== matlab function proxy/Generate SchunkCommands /Index Finger/New Version/Index New Pose Estimation  ==
  data: Sensors input; pose output; Finger input
function pose = fcn(Sensors, Finger)
%#codegen


lx = Sensors (1);
qB = Sensors (2);

LLM =  Finger(1);   
LIIp = Finger(2);
% LJJp = Finger(3);

% LLM = 50; %fing length
% LIIp = 23.8; %fing width,

%#codegen
LKN = 147.669; %%135.6320;


% LAB =  12.7;
LBC =  43;
LCD =  9;
LDE =  40;
LEF =  27;
LBH =  37; 
LGH =  86;
LGF =  46;
LEJ =  39;
LCI =  16;
% LKL =  24.2;
LKB =  35;
LBK = LKB;
LA2A1 = 13;
LA2B = 16.78;
xL = -10 ;  
offset = 1.8;
yL = - (LIIp - offset);

% LKNx = 134.8;
% LKNy = 15;

% LKLx = -10;
% LKLy = -23;

% qKL = 2.0344;
% qKL = 114.4 * pi / 180; %2.8501;
qKN = 11.5 * pi/180; %%0.1108;

lact = 123; %%117.77;
% lact2 = 13;
% lact3 = 12.5;
% LNO = lact;

LKH = LKB + LBH;

LDF = LDE + LEF;

LBD = LBC + LCD;

LA1N = lx + lact;

LA2K = sqrt(LA2B^2 + LKB^2 - 2*LA2B*LKB*cos(qB));

% qA2
qA2 = my_acos((- LBK^2 + LA2B^2 + LA2K^2)/(2 * LA2B * LA2K));


LA1K = sqrt(LA2A1^2 + LA2K^2 - 2*LA2A1*LA2K*cos(115 * pi/180 - qA2));

    qN = abs(my_acos(((- LA1K^2 + LA1N^2 + LKN^2)/(2*LA1N*LKN)))) - qKN;
    
    xK1 = ((-LA2B^2 + LA2K^2 + LKB^2)/(2*LA2K*LKB));
    
    
    xK2 = (-LA1N^2 + LA1K^2 + LKN^2)/(2*LA1K*LKN);
    xK3 = (-LA2A1^2 + LA2K^2 + LA1K^2)/(2*LA2K*LA1K);
    
    if my_acos(xK1) >= 0
        qK1 = abs(my_acos(xK1));
    else 
        qK1 = abs(my_acos(xK1)) + pi/2;
    end
    
    if my_acos(xK2) >= 0
        qK2 = abs(my_acos(xK2));
    else 
        qK2 = abs(my_acos(xK2)) + pi/2;
    end
    
    if my_acos(xK3) >= 0
        qK3 = abs(my_acos(xK3));
    else 
        qK3 = abs(my_acos(xK3)) + pi/2;
    end
    
        qK = pi - (qK1 + qK2 + qK3 + qKN);
    
xB = - LKB * cos(qK);  yB = LKB * sin(qK);
xH = - LKH * cos(qK);  yH = LKH * sin(qK);
xG = xH - LGH*sin(qK);  yG = yH - LGH*cos(qK);

xC = xB - LBC*cos(qB - qK); yC = yB - LBC * sin(qB - qK);
xD = xC - LCD*cos(qB - qK);   yD = yC - LCD*sin(qB - qK);
xI = xC + LCI * sin(qB - qK);   yI = yC - LCI * cos(qB - qK);

LLI = sqrt((xI - xL)^2 + (yI - yL)^2);

    c1 = sqrt(LLI^2 - LIIp^2);
    
    xj1 = (-LIIp^2 + LLI^2 + c1^2)/(2*c1*LLI);
    
    if my_acos(xj1) >= 0
        qj1 = abs(my_acos(xj1));
    else 
        qj1 = abs(my_acos(xj1)) + pi/2;
    end
    
    qo1 = qj1 + atan((yL - yI)/(xL - xI));



LHD = sqrt((xH - xD)^2 + (yH - yD)^2);

LDG = sqrt((xG - xD)^2 + (yG - yD)^2);


    xG1 = (-LHD^2 + LDG^2 + LGH^2)/(2*LDG*LGH);
    xG2 = (-LDF^2 + LDG^2 + LGF^2)/(2*LDG*LGF);
    
    if my_acos(xG1) >= 0
        qG1 = abs(my_acos(xG1));
    else 
        qG1 = abs(my_acos(xG1)) + pi/2;
    end
    
    if my_acos(xG2) >= 0
        qG2 = abs(my_acos(xG2));
    else 
        qG2 = abs(my_acos(xG2)) + pi/2;
    end

    qG = pi - (qG1 + qG2);
    


xM = xL - LLM*cos(qo1); yM = yL - LLM*sin(qo1);



    xD1 = (-LGH^2 + LHD^2 + LDG^2)/(2*LHD*LDG);
    xD2 = (-LGF^2 + LDG^2 + LDF^2)/(2*LDG*LDF);
    xD3 = (-LBH^2 + LHD^2 + LBD^2)/(2*LHD*LBD);
    
    if my_acos(xD1) >= 0
        qD1 = abs(my_acos(xD1));
    else 
        qD1 = abs(my_acos(xD1)) + pi/2;
    end
    
    if my_acos(xD2) >= 0
        qD2 = abs(my_acos(xD2));
    else 
        qD2 = abs(my_acos(xD2)) + pi/2;
    end

    if my_acos(xD3) >= 0
        qD3 = abs(my_acos(xD3));
    else 
        qD3 = abs(my_acos(xD3)) + pi/2;
    end

    qD = pi - (qD1 + qD2 + qD3);
    
xE = xD - LDE*cos(qB - qD - qK);
yE = yD - LDE*sin(qB - qD - qK);
xJ = xE + LEJ*sin(qB - qD - qK);  
yJ = yE - LEJ*cos(qB - qD - qK);


LJM = sqrt((xJ - xM)^2 + (yJ - yM)^2);

% if LJM^2 - LIIp^2 > 0
    c2 = sqrt(LJM^2 - LIIp^2);
% else
%     c2 = sqrt(-LJM^2 + LIIp^2);
% end

    xj2 = (-LIIp^2 + LJM^2 + c2^2)/(2*c2*LJM);
    
    if my_acos(xj2)>= 0
        qj2 = abs(my_acos(xj2));
    else 
        qj2 = abs(my_acos(xj2)) + pi/2;
    end 
    
    if (xJ - xM)<=0
        qj3 = atan((yJ - yM)/(xJ - xM));
    else
        qj3 = pi + atan((yJ - yM)/(xJ - xM));
    end
    
    qo2 = qj2 + qj3 - qo1;
% if (qo1 < 0)
%     qo1o = jold(1);
% else 
%     qo1o = qo1;
% end
% 
% if (qo2 < 0)
%     qo2o = jold(2);
% else 
%     qo2o = qo2;
% end

    pose = [qo1; qo2; qK; qD; qG; qN; c1; c2 ];
%     dene = [deneK1; deneK2; deneJ1; deneJ2; deneG1; deneG2; deneD1; deneD2; deneD3; deneJ3; deneJ4];
%     
end
%%%
function a = my_acos(b)
    if b < -1
        a = single(-1)
    else
        if b > 1
            a = single(1)
        else
            a = b;
        end
    end
end

== matlab function proxy/Generate SchunkCommands /Index Finger/Old Version/Pose Generator/Pose ==
  data: u input; y output; measurements input
function y  = fcn(u, measurements)
%#codegen
LKN =  135.6320;

LAB =  18;
LBC =  43;
LCD =  9;
LDE =  40;
LEF =  27;
LBH =  37; 
LGH =  86;
LGF =  46;
LEJ =  39;
LCI =  16;
lact = 117.77;
% LNO = lact;

offset = 3;
xL_mag = 10;

LKB =  35;

LKH = LKB + LBH;
LDF = LDE + LEF;
LBD = LBC + LCD;

% LKL =  22.3607;
% LKNx = 134.8;
% LKNy = 15;
% 
% LKLx = -10;
% LKLy = -23;

qKL = 2.0344;
% qKL = 2.8501
% 
%%%%%%%%%%% qKL possibilities
 qKN = 0.1108;
%  qKN = 0.1767;  %% cetvelle olctugume gore cikan aci
% qKN = 0.2653;  %% CAD olcumlerine force sensor farikin ekledigimde cikan aci 


%%%%%%%%%%% finger

% LIIp = 7; %fing width phalange 1
% LJJp = 4; %fing width phalange 2
% LLM =  48;   %fing length
% offset = 3;

LIIp = measurements(1);
LJJp = LIIp;
LLM = measurements(2);


% LIIp = 7;
% LJJp = LIIp;
% LLM = 50;
% offset = 3;
% xL_mag = 10;

% xL = -3;
xL = -xL_mag;  
% xL = -10;
yL = -(LIIp + offset);

lx = u(1);
qB = u(2);

atemp = LAB^2 + LKB^2 - 2*LAB*LKB*cos(qB);
if atemp < 0
    fprintf('errore LAK \n');
    atemp = single(1); % Non 0 se no i denominatori vanno a 0
end
LAK = sqrt(atemp);

if abs((- LAK^2 + (lx+lact)^2 + LKN^2)/(2*(lx+lact)*LKN)) > 1
    fprintf('errore qN');
    qN = single(0);
else
    qN = abs(acos(((- LAK^2 + (lx+lact)^2 + LKN^2)/(2*(lx+lact)*LKN)))) - qKN;
end

xK1 = (-LAB^2 + LAK^2 + LKB^2)/(2*LAK*LKB);
xK2 = (-(lx+lact)^2 + LAK^2 + LKN^2)/(2*LAK*LKN);

%% qK1
if abs(xK1) > 1
    fprintf('errore qK1 \n');
    qK1 = single(0);
else
    if acos(xK1) >= 0
        qK1 = abs(acos(xK1));
    else 
        qK1 = abs(acos(xK1)) + pi/2;
    end
end

%% qK2
if abs(xK2) > 1
    fprintf('errore gK2 \n');
    qK2 = single(0);
else
    if acos(xK2) >= 0
        qK2 = abs(acos(xK2));
    else 
        qK2 = abs(acos(xK2)) + pi/2;
    end
end

    
qK = pi - ( qK1 + qK2 + qKN);
    
xB = - LKB * cos(qK);  yB = LKB * sin(qK);
xH = - LKH * cos(qK);  yH = LKH * sin(qK);
xG = xH - LGH*sin(qK);  yG = yH - LGH*cos(qK);

xC = xB - LBC*cos(qB - qK); yC = yB - LBC * sin(qB - qK);
xD = xC - LCD*cos(qB - qK);   yD = yC - LCD*sin(qB - qK);
xI = xC + LCI * sin(qB - qK);   yI = yC - LCI * cos(qB - qK);

LLI = sqrt((xI - xL)^2 + (yI - yL)^2);
% LLI = 1;

%% c1
atemp = LLI^2 - LIIp^2;
if atemp < 0
    fprintf('errore c1 \n');
    atemp = single(0);
end
c1 = sqrt(atemp);


xj1 = (-LIIp^2 + LLI^2 + c1^2)/(2*c1*LLI);

%% qj1
if abs(xj1) > 1
    fprintf('errore qj1 \n');
    qj1 = single(0);
else
    if acos(xj1) >= 0
        qj1 = abs(acos(xj1));
    else 
        qj1 = abs(acos(xj1)) + pi/2;
    end
end
% qj1 = acos(xj1);
    
qo1_c = qj1 + atan((yL - yI)/(xL - xI));

%%%% SATURATION:
if qo1_c<= 0
    qo1 = abs(qo1_c);
else
    qo1 = qo1_c;
end


    
   
LHD = sqrt((xH - xD)^2 + (yH - yD)^2);
LDG = sqrt((xG - xD)^2 + (yG - yD)^2);
% LHD = 1; LDG = 1;

xG1 = (-LHD^2 + LDG^2 + LGH^2)/(2*LDG*LGH);
xG2 = (-LDF^2 + LDG^2 + LGF^2)/(2*LDG*LGF);

%% qG1
if abs(xG1) > 1
    fprintf('errore qG1 \n')
    qG1 = single(0);
else
    if acos(xG1) >= 0
        qG1 = abs(acos(xG1));
    else 
        qG1 = abs(acos(xG1)) + pi/2;
    end
end

% qG1 = acos(xG1);

%% qG2
if abs(xG2) > 1
    fprintf('errore qG2 \n');
    qG2 = single(0);
else
    if acos(xG2) >= 0
        qG2 = abs(acos(xG2));
    else 
        qG2 = abs(acos(xG2)) + pi/2;
    end
end
% qG2 = acos(xG2);

qG = pi - (qG1 + qG2);

xM = xL - LLM*cos(qo1); yM = yL - LLM*sin(qo1);

xD1 = (-LGH^2 + LHD^2 + LDG^2)/(2*LHD*LDG);
xD2 = (-LGF^2 + LDG^2 + LDF^2)/(2*LDG*LDF);
xD3 = (-LBH^2 + LHD^2 + LBD^2)/(2*LHD*LBD);

%% qD1
if abs(xD1) > 1
    fprintf('errore qD1');
    qD1 = single(0);
else
    if acos(xD1) >= 0
        qD1 = abs(acos(xD1));
    else 
        qD1 = abs(acos(xD1)) + pi/2;
    end
end

%     qD1 = acos(xD1);
%% qD2
if abs(xD2) > 1
    fprintf('errore qD2 \n');
    qD2 = single(0);
else
    if acos(xD2) >= 0
        qD2 = abs(acos(xD2));
    else 
        qD2 = abs(acos(xD2)) + pi/2;
    end
end
% qD2 = acos(xD2);

%% qD3
if abs(xD3) > 1
    fprintf('errore qD3 \n');
    qD3 = single(0);
else
    if acos(xD3) >= 0
        qD3 = abs(acos(xD3));
    else 
        qD3 = abs(acos(xD3)) + pi/2;
    end
end
%     qD3 = acos(xD3);

qD = pi - (qD1 + qD2 + qD3);


xE = xD - LDE*cos(qB - qD - qK);
yE = yD - LDE*sin(qB - qD - qK);
xJ = xE + LEJ*sin(qB - qD - qK);  
yJ = yE - LEJ*cos(qB - qD - qK);

LJM = sqrt((xJ - xM)^2 + (yJ - yM)^2);

atemp = LJM^2 - LJJp^2;
if atemp < 0
    fprintf('errore c2');
    c2 = single(0);
else
    c2 = sqrt(atemp);
end
xj2 = (-LIIp^2 + LJM^2 + c2^2)/(2*c2*LJM);

%% qj2
if abs(xj2) > 1
    fprintf('errore qj2 \n');
    qj2 = single(0);
else
    if acos(xj2) >= 0
        qj2 = abs(acos(xj2));
    else 
        qj2 = abs(acos(xj2)) + pi/2;
    end 
end
% qj2 = acos(xj2);

 if (xJ - xM)<=0
    qj3 = atan((yJ - yM)/(xJ - xM));
else
    qj3 = pi + atan((yJ - yM)/(xJ - xM));
 end


qo2d = qj2 + qj3 - qo1;

if qo2d <= - pi/2
    %Sostituito con la dicitura del codice
    %qo2a = 2*pi + qo2d;
    qo2 = (2*pi + qo2d);% * 0.7;
else 
    %Sostituito con la dicitura del codice
    %qo2a = qo2d; 
    qo2 = (qo2d);% * 0.7; 
end

% 
% if qo2a <= 0
%     qo2 = abs(qo2a);
% else 
%     qo2 = qo2a;
% end


%     if qo2 <= 0
%         qo2 = 0;
%     else if qo2 >= 2.1
%             qo2 = 2.1;
%         else 
%             qo2 = qo2;
%         end
%     end

y = [qo1; qo2; qK; qD; qG; qN; c1; c2];
%     more = [qj2; qj3; xJ - xM; yJ - yM];
%     lengths = [LLM; LIIp];

== matlab function proxy/Generate SchunkCommands /Middle Finger/MATLAB Function2 ==
  data: cons input; sens input; y output; enab input
function y = fcn(cons, sens, enab)

if (enab == 0)
    use = cons;
else 
    use = sens;
end

y = use;

== matlab function proxy/Generate SchunkCommands /Middle Finger/MATLAB Function3 ==
  data: u input; y output; measurements input
function y  = fcn(u, measurements)
%#codegen
LKN =  135.6320;

LAB =  18;
LBC =  43;
LCD =  9;
LDE =  40;
LEF =  27;
LBH =  37; 
LGH =  86;
LGF =  46;
LEJ =  39;
LCI =  16;
lact = 117.77;
% LNO = lact;

offset = 3;
xL_mag = 10;

LKB =  35;

LKH = LKB + LBH;
LDF = LDE + LEF;
LBD = LBC + LCD;

% LKL =  22.3607;
% LKNx = 134.8;
% LKNy = 15;
% 
% LKLx = -10;
% LKLy = -23;

qKL = 2.0344;
% qKL = 2.8501
% 
%%%%%%%%%%% qKL possibilities
 qKN = 0.1108;
%  qKN = 0.1767;  %% cetvelle olctugume gore cikan aci
% qKN = 0.2653;  %% CAD olcumlerine force sensor farikin ekledigimde cikan aci 


%%%%%%%%%%% finger

% LIIp = 7; %fing width phalange 1
% LJJp = 4; %fing width phalange 2
% LLM =  48;   %fing length
% offset = 3;

LIIp = measurements(1);
LJJp = LIIp;
LLM = measurements(2);


% LIIp = 7;
% LJJp = LIIp;
% LLM = 50;
% offset = 3;
% xL_mag = 10;

% xL = -3;
xL = -xL_mag;  
% xL = -10;
yL = -(LIIp + offset);

lx = u(1);
qB = u(2);

atemp = LAB^2 + LKB^2 - 2*LAB*LKB*cos(qB);
if atemp < 0
    fprintf('errore LAK \n');
    atemp = single(1); % Non 0 se no i denominatori vanno a 0
end
LAK = sqrt(atemp);

if abs((- LAK^2 + (lx+lact)^2 + LKN^2)/(2*(lx+lact)*LKN)) > 1
    fprintf('errore qN');
    qN = single(0);
else
    qN = abs(acos(((- LAK^2 + (lx+lact)^2 + LKN^2)/(2*(lx+lact)*LKN)))) - qKN;
end

xK1 = (-LAB^2 + LAK^2 + LKB^2)/(2*LAK*LKB);
xK2 = (-(lx+lact)^2 + LAK^2 + LKN^2)/(2*LAK*LKN);

%% qK1
if abs(xK1) > 1
    fprintf('errore qK1 \n');
    qK1 = single(0);
else
    if acos(xK1) >= 0
        qK1 = abs(acos(xK1));
    else 
        qK1 = abs(acos(xK1)) + pi/2;
    end
end

%% qK2
if abs(xK2) > 1
    fprintf('errore gK2 \n');
    qK2 = single(0);
else
    if acos(xK2) >= 0
        qK2 = abs(acos(xK2));
    else 
        qK2 = abs(acos(xK2)) + pi/2;
    end
end

    
qK = pi - ( qK1 + qK2 + qKN);
    
xB = - LKB * cos(qK);  yB = LKB * sin(qK);
xH = - LKH * cos(qK);  yH = LKH * sin(qK);
xG = xH - LGH*sin(qK);  yG = yH - LGH*cos(qK);

xC = xB - LBC*cos(qB - qK); yC = yB - LBC * sin(qB - qK);
xD = xC - LCD*cos(qB - qK);   yD = yC - LCD*sin(qB - qK);
xI = xC + LCI * sin(qB - qK);   yI = yC - LCI * cos(qB - qK);

LLI = sqrt((xI - xL)^2 + (yI - yL)^2);
% LLI = 1;

%% c1
atemp = LLI^2 - LIIp^2;
if atemp < 0
    fprintf('errore c1 \n');
    atemp = single(0);
end
c1 = sqrt(atemp);


xj1 = (-LIIp^2 + LLI^2 + c1^2)/(2*c1*LLI);

%% qj1
if abs(xj1) > 1
    fprintf('errore qj1 \n');
    qj1 = single(0);
else
    if acos(xj1) >= 0
        qj1 = abs(acos(xj1));
    else 
        qj1 = abs(acos(xj1)) + pi/2;
    end
end
% qj1 = acos(xj1);
    
qo1_c = qj1 + atan((yL - yI)/(xL - xI));

%%%% SATURATION:
if qo1_c<= 0
    qo1 = abs(qo1_c);
else
    qo1 = qo1_c;
end


    
   
LHD = sqrt((xH - xD)^2 + (yH - yD)^2);
LDG = sqrt((xG - xD)^2 + (yG - yD)^2);
% LHD = 1; LDG = 1;

xG1 = (-LHD^2 + LDG^2 + LGH^2)/(2*LDG*LGH);
xG2 = (-LDF^2 + LDG^2 + LGF^2)/(2*LDG*LGF);

%% qG1
if abs(xG1) > 1
    fprintf('errore qG1 \n')
    qG1 = single(0);
else
    if acos(xG1) >= 0
        qG1 = abs(acos(xG1));
    else 
        qG1 = abs(acos(xG1)) + pi/2;
    end
end

% qG1 = acos(xG1);

%% qG2
if abs(xG2) > 1
    fprintf('errore qG2 \n');
    qG2 = single(0);
else
    if acos(xG2) >= 0
        qG2 = abs(acos(xG2));
    else 
        qG2 = abs(acos(xG2)) + pi/2;
    end
end
% qG2 = acos(xG2);

qG = pi - (qG1 + qG2);

xM = xL - LLM*cos(qo1); yM = yL - LLM*sin(qo1);

xD1 = (-LGH^2 + LHD^2 + LDG^2)/(2*LHD*LDG);
xD2 = (-LGF^2 + LDG^2 + LDF^2)/(2*LDG*LDF);
xD3 = (-LBH^2 + LHD^2 + LBD^2)/(2*LHD*LBD);

%% qD1
if abs(xD1) > 1
    fprintf('errore qD1');
    qD1 = single(0);
else
    if acos(xD1) >= 0
        qD1 = abs(acos(xD1));
    else 
        qD1 = abs(acos(xD1)) + pi/2;
    end
end

%     qD1 = acos(xD1);
%% qD2
if abs(xD2) > 1
    fprintf('errore qD2 \n');
    qD2 = single(0);
else
    if acos(xD2) >= 0
        qD2 = abs(acos(xD2));
    else 
        qD2 = abs(acos(xD2)) + pi/2;
    end
end
% qD2 = acos(xD2);

%% qD3
if abs(xD3) > 1
    fprintf('errore qD3 \n');
    qD3 = single(0);
else
    if acos(xD3) >= 0
        qD3 = abs(acos(xD3));
    else 
        qD3 = abs(acos(xD3)) + pi/2;
    end
end
%     qD3 = acos(xD3);

qD = pi - (qD1 + qD2 + qD3);


xE = xD - LDE*cos(qB - qD - qK);
yE = yD - LDE*sin(qB - qD - qK);
xJ = xE + LEJ*sin(qB - qD - qK);  
yJ = yE - LEJ*cos(qB - qD - qK);

LJM = sqrt((xJ - xM)^2 + (yJ - yM)^2);

atemp = LJM^2 - LJJp^2;
if atemp < 0
    fprintf('errore c2');
    c2 = single(0);
else
    c2 = sqrt(atemp);
end
xj2 = (-LIIp^2 + LJM^2 + c2^2)/(2*c2*LJM);

%% qj2
if abs(xj2) > 1
    fprintf('errore qj2 \n');
    qj2 = single(0);
else
    if acos(xj2) >= 0
        qj2 = abs(acos(xj2));
    else 
        qj2 = abs(acos(xj2)) + pi/2;
    end 
end
% qj2 = acos(xj2);

 if (xJ - xM)<=0
    qj3 = atan((yJ - yM)/(xJ - xM));
else
    qj3 = pi + atan((yJ - yM)/(xJ - xM));
 end


qo2d = qj2 + qj3 - qo1;

if qo2d <= - pi/2
    %Sostituito con la dicitura del codice
    %qo2a = 2*pi + qo2d;
    qo2 = (2*pi + qo2d);% * 0.7;
else 
    %Sostituito con la dicitura del codice
    %qo2a = qo2d; 
    qo2 = (qo2d);% * 0.7; 
end

% 
% if qo2a <= 0
%     qo2 = abs(qo2a);
% else 
%     qo2 = qo2a;
% end


%     if qo2 <= 0
%         qo2 = 0;
%     else if qo2 >= 2.1
%             qo2 = 2.1;
%         else 
%             qo2 = qo2;
%         end
%     end

y = [qo1; qo2; qK; qD; qG; qN; c1; c2];
%     more = [qj2; qj3; xJ - xM; yJ - yM];
%     lengths = [LLM; LIIp];
